simulink model "exampleModel_PyTorch_import"  (R2026a)
settings: Solver=FixedStepDiscrete  StopTime=steps  FixedStep=1
libraries: deeplib x1
settings Model: Creator=jianghaw  LastModifiedBy=wenzheli
settings SFSimCC: SimTargetLang=C++

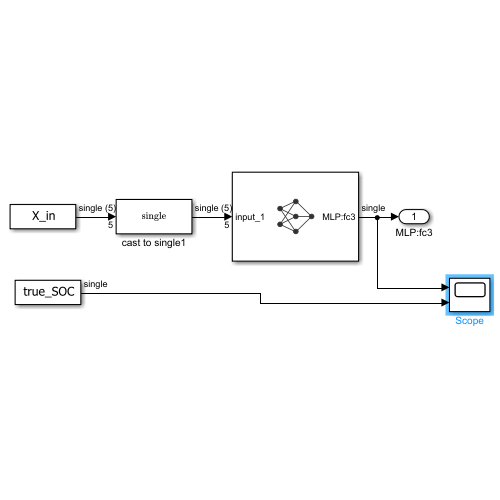
[thumbnail: Simulink's stored preview of the top-level diagram]
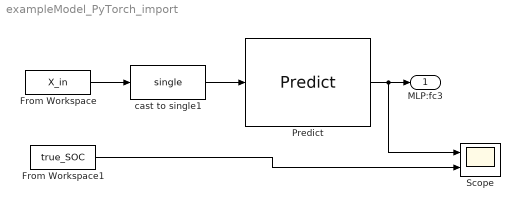
== system exampleModel_PyTorch_import ==
  From Workspace : FromWorkspace  VariableName=X_in
  From Workspace1 : FromWorkspace  VariableName=true_SOC
  Predict : deeplib/Predict  Network=Network from MAT-file  NetworkFunction=squeezenet  NetworkFilePath=netPyTorchMLP.mat  MiniBatchSize=128  SimulateUsing=Auto mode  InputDataFormats={ 'input_1', 'UU' }  Predictions=on  Activations={}  ForceInterpretedSim=off  EnableDLNetwork=on  LastKnownNetworkFilePath='netPyTorchMLP.mat'  LastKnownNetworkTimeStamp=740109.56708333338610827922821044921875
  Scope : Scope  NumInputPorts=2
      settings: ActiveDisplayYMinimum=0.14075001701712611  ActiveDisplayYMaximum=1.1110612191259861
  cast to single1 : DataTypeConversion  OutDataTypeStr=single  SaturateOnIntegerOverflow=off  RndMeth=Floor
  MLP:fc3 : Outport
  wires:
  cast to single1/1 -> Predict/1
  Predict/1 -> Scope/1, MLP:fc3/1
  From Workspace/1 -> cast to single1/1
  From Workspace1/1 -> Scope/2
